simulink model "plant_adaptive_switching"  (R2024a)
settings: Solver=VariableStepAuto  StartTime=0.0  StopTime=10.0  RelTol=1e-3
values from neighbouring files (symbols this model uses):
  a1 = 0.22    [CA1_params.m]
  a1_new = 20.4    [CA1_params.m]
  a2 = 6.1    [CA1_params.m]
  a2_new = 6.4    [CA1_params.m]
  b0 = -0.5    [CA1_params.m]
  b0_new = -2    [CA1_params.m]
  b1 = -1    [CA1_params.m]
  b1_new = -5    [CA1_params.m]
settings Model: Creator=john  LastModifiedBy=john

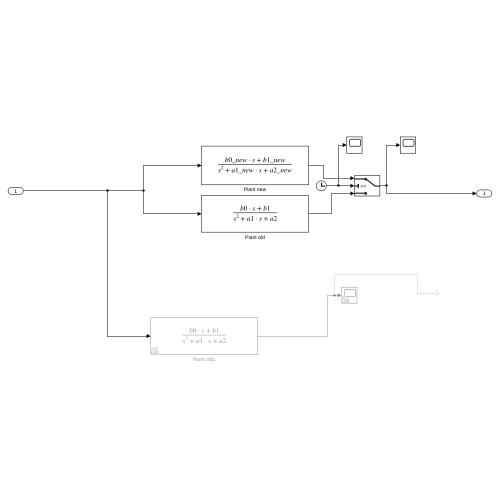
[thumbnail: Simulink's stored preview of the top-level diagram]
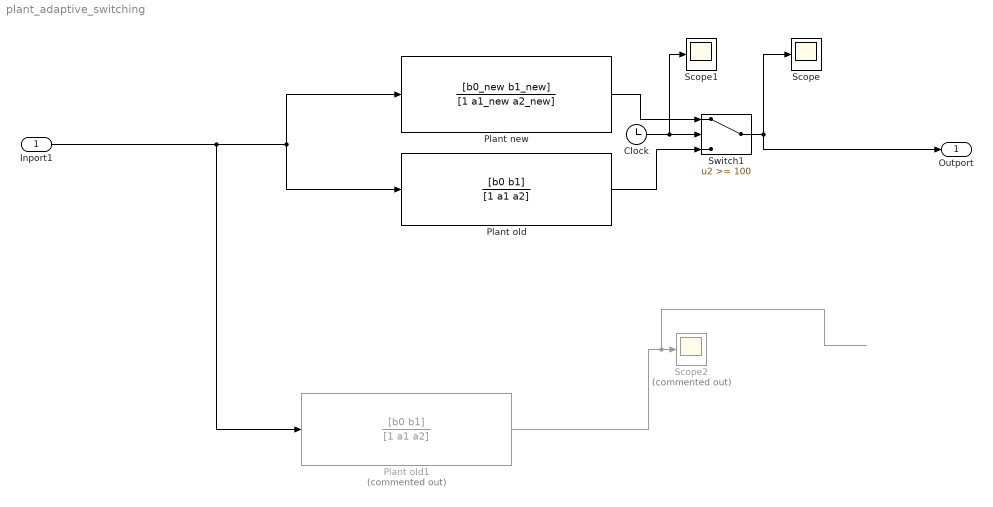
== system plant_adaptive_switching ==
  Inport1 : Inport
  Clock : Clock
  Plant new : TransferFcn  Numerator=[b0_new b1_new]  Denominator=[1 a1_new a2_new]
  Plant old : TransferFcn  Numerator=[b0 b1]  Denominator=[1 a1 a2]
  Plant old1 : TransferFcn  Commented=on  Numerator=[b0 b1]  Denominator=[1 a1 a2]
  Scope : Scope
  Scope1 : Scope
  Scope2 : Scope  Commented=on
  Switch1 : Switch  Threshold=100  SaturateOnIntegerOverflow=off  InputSameDT=off
  Outport : Outport
  wires:
  Plant old/1 -> Switch1/3
  Clock/1 -> Scope1/1, Switch1/2
  Plant new/1 -> Switch1/1
  Switch1/1 -> Outport/1, Scope/1
  Inport1/1 -> Plant old1/1, Plant new/1, Plant old/1
  Plant old1/1 -> Scope2/1
